simulink model "Q2B"  (R2021b)
settings: Solver=ode23s  StartTime=0.0  StopTime=1  MaxStep=1e-4  MinStep=1e-5  RelTol=1e-3  EnableMultiTasking=on
libraries: spsabctodq0Lib x1
settings Model: Creator=WQJ  LastModifiedBy=ds
settings SolverCC: AlgebraicLoopSolver=TrustRegion
settings DataIOCC: LimitDataPoints=on  SaveFormat=Array  SignalLoggingSaveFormat=ModelDataLogs  ReturnWorkspaceOutputs=off
settings OptimizationCC: InitFltsAndDblsToZero=on  LifeSpan=inf
settings DebuggingCC: SaveWithParameterizedLinksMsg=none  UnderspecifiedInitializationDetection=Classic  MergeDetectMultiDrivingBlocksExec=none  SignalResolutionControl=TryResolveAllWithWarning  MultiTaskDSMMsg=warning  MultiTaskCondExecSysMsg=none  FcnCallInpInsideContextMsg=warning  SFUnexpectedBacktrackingDiag=warning  SFNoUnconditionalDefaultTransitionDiag=warning  SFExecutionAtInitializationDiag=none  SFMachineParentedDataDiag=warning  ArithmeticOperatorsInVariantConditions=warning
settings HardwareCC: ProdBitPerPointer=32  ProdBitPerSizeT=32  ProdBitPerPtrDiffT=32  ProdLargestAtomicFloat=None  ProdIntDivRoundTo=Undefined  ProdEndianess=Unspecified  ProdWordSize=32  ProdHWDeviceType=32-bit Generic  TargetUnknown=on
settings ModelReferenceCC: PropagateSignalLabelsOutOfModel=off
settings CodeAppCC: StateflowObjectComments=on
settings GRTTargetCC: TargetFcnLib=ansi_tfl_tmw.mat  TargetLangStandard=C89/C90 (ANSI)  CombineOutputUpdateFcns=off  GRTInterface=on
settings ConfigComp: CovMetricSettings=dw  CovSaveCumulativeToWorkspaceVar=on  CovSaveSingleToWorkspaceVar=on

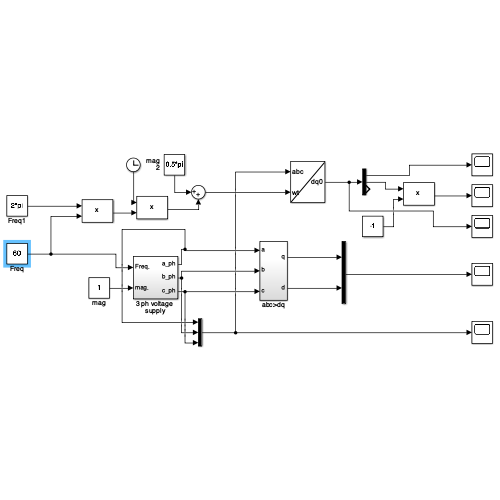
[thumbnail: Simulink's stored preview of the top-level diagram]
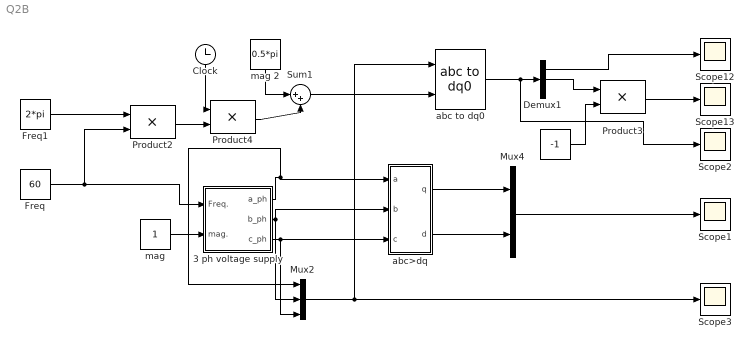
== system Q2B ==
  " " : Constant  Value=-1
  3 ph voltage supply : Subsystem
  Clock : Clock
  Demux1 : Demux  Outputs=3
  Freq : Constant  Value=60
  Freq1 : Constant  Value=2*pi
  Mux2 : Mux  Inputs=3
  Mux4 : Mux  Inputs=2
  Product2 : Product  SaturateOnIntegerOverflow=on  OutDataTypeStr=Inherit: Same as first input
  Product3 : Product  SaturateOnIntegerOverflow=on  OutDataTypeStr=Inherit: Same as first input
  Product4 : Product  SaturateOnIntegerOverflow=on  OutDataTypeStr=Inherit: Same as first input
  Scope{1..3,12..13} (5 alike) : Scope
  Sum1 : Sum  Inputs=|++  SaturateOnIntegerOverflow=on
  abc to dq0 : spsabctodq0Lib/abc to dq0  Alignment=Aligned with phase A axis
  abc>dq : Subsystem
  "mag " : Constant
  mag 2 : Constant  Value=0.5*pi
  wires:
  Freq/1 -> Product2/2, 3 ph voltage supply/1(Freq.)
  "mag "/1 -> 3 ph voltage supply/2(mag.)
  3 ph voltage supply/1(a_ph) -> Mux2/1, abc>dq/1(a)
  3 ph voltage supply/2(b_ph) -> abc>dq/2(b), Mux2/2
  3 ph voltage supply/3(c_ph) -> abc>dq/3(c), Mux2/3
  abc>dq/1(q) -> Mux4/1
  abc>dq/2(d) -> Mux4/2
  Mux2/1 -> Scope3/1, abc to dq0/1
  Mux4/1 -> Scope1/1
  Freq1/1 -> Product2/1
  Clock/1 -> Product4/1
  Product2/1 -> Product4/2
  abc to dq0/1 -> Scope2/1, Demux1/1
  Sum1/1 -> abc to dq0/2
  Product4/1 -> Sum1/2
  Demux1/2 -> Product3/1
  Demux1/1 -> Scope12/1
  " "/1 -> Product3/2
  Product3/1 -> Scope13/1
  mag 2/1 -> Sum1/1

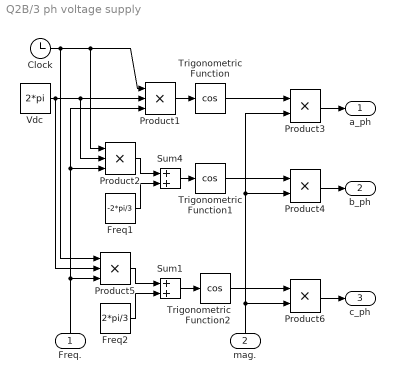
== system Q2B/3 ph voltage supply ==
  Freq. : Inport
  mag. : Inport  Port=2
  Clock : Clock
  Freq1 : Constant  Value=-2*pi/3
  Freq2 : Constant  Value=2*pi/3
  Product1 : Product  Inputs=3  RndMeth=Zero
  Product2 : Product  Inputs=3  RndMeth=Zero
  Product3 : Product  RndMeth=Zero
  Product4 : Product  RndMeth=Zero
  Product5 : Product  Inputs=3  RndMeth=Zero
  Product6 : Product  RndMeth=Zero
  Sum1 : Sum  InputSameDT=on  SaturateOnIntegerOverflow=on  OutDataTypeStr=Inherit: Same as first input
  Sum4 : Sum  InputSameDT=on  SaturateOnIntegerOverflow=on  OutDataTypeStr=Inherit: Same as first input
  Trigonometric Function : Trigonometry  Operator=cos
  Trigonometric Function1 : Trigonometry  Operator=cos
  Trigonometric Function2 : Trigonometry  Operator=cos
  Vdc : Constant  Value=2*pi
  a_ph : Outport
  b_ph : Outport  Port=2
  c_ph : Outport  Port=3
  wires:
  Product1/1 -> Trigonometric Function/1
  Vdc/1 -> Product1/2, Product2/2, Product5/2
  Clock/1 -> Product1/1, Product2/1, Product5/1
  Freq./1 -> Product5/3, Product2/3, Product1/3
  Sum4/1 -> Trigonometric Function1/1
  Product2/1 -> Sum4/1
  Freq1/1 -> Sum4/2
  Trigonometric Function1/1 -> Product4/1
  Trigonometric Function/1 -> Product3/1
  Sum1/1 -> Trigonometric Function2/1
  Product5/1 -> Sum1/1
  Freq2/1 -> Sum1/2
  Trigonometric Function2/1 -> Product6/1
  mag./1 -> Product6/2, Product4/2, Product3/2
  Product3/1 -> a_ph/1
  Product4/1 -> b_ph/1
  Product6/1 -> c_ph/1

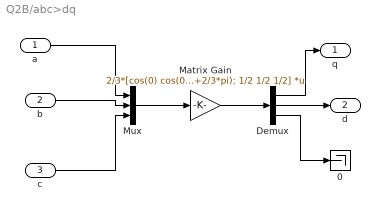
== system Q2B/abc>dq ==
  a : Inport
  b : Inport  Port=2
  c : Inport  Port=3
  0 : Terminator
  Demux : Demux  Outputs=3
      settings: DisplayOption=none
  Matrix Gain : Gain  Gain=2/3*[cos(0) cos(0-2/3*pi) cos(0+2/3*pi);-sin(0) -sin(0-2/3*pi) -sin(0+2/3*pi); 1/2 1/2 1/2]  Multiplication=Matrix(K*u)  SaturateOnIntegerOverflow=on  OutDataTypeStr=Inherit: Same as input  ParamDataTypeStr=Inherit: Same as input
  Mux : Mux  Inputs=3
  q : Outport
  d : Outport  Port=2
  wires:
  a/1 -> Mux/1
  b/1 -> Mux/2
  c/1 -> Mux/3
  Demux/1 -> q/1
  Demux/2 -> d/1
  Mux/1 -> Matrix Gain/1
  Matrix Gain/1 -> Demux/1
  Demux/3 -> 0/1
